simulink model "SegmentsDisplays"  (R2020b)
settings: Solver=FixedStepAuto  StartTime=0.0  StopTime=Inf  RelTol=1e-3  SampleTimeConstraint=STIndependent
undefined symbols (not defined in the file): DISPLAY_REGISTER_1, DISPLAY_REGISTER_2, DISPLAY_REGISTER_3
Description:
  | % Copyright 2019 The MathWorks, Inc.
settings Model: DataDictionary=Parameters.sldd  EnableAccessToBaseWorkspace=off  EnablePacing=on  Creator=sdupertu  LastModifiedBy=sebas
settings DataIOCC: SaveOutput=off  SaveTime=off
settings OptimizationCC: DefaultParameterBehavior=Inlined  EnhancedBackFolding=on  PassReuseOutputArgsAs=Individual arguments  OptimizeBlockOrder=speed  DifferentSizesBufferReuse=on  OptimizationCustomize=off  EfficientTunableParamExpr=on
settings DebuggingCC: ParameterTunabilityLossMsg=error  PregeneratedLibrarySubsystemCodeDiagnostic=none  ArithmeticOperatorsInVariantConditions=warning
settings ModelReferenceCC: EnableParallelModelReferenceBuilds=on
settings SFSimCC: SimUseLocalCustomCode=off  MATLABDynamicMemAlloc=off  CustomCodeUndefinedFunction=UseInterfaceOnly
settings RTWCC: Description=Embedded Coder  SystemTargetFile=ert.tlc  TemplateMakefile=ert_default_tmf  GenerateReport=on  RTWUseLocalCustomCode=off  IncludeHyperlinkInReport=on  LaunchReport=on  GenerateTraceInfo=on  GenerateTraceReport=on  GenerateTraceReportSl=on  GenerateTraceReportSf=on  GenerateTraceReportEml=on  GenerateWebview=on  GenerateCodeMetricsReport=on
settings CodeAppCC: ForceParamTrailComments=on  IgnoreCustomStorageClasses=off  MaxIdLength=61  OperatorAnnotations=on  SimulinkDataObjDesc=on  SFDataObjDesc=on  InsertBlockDesc=on
settings ERTTargetCC: TargetLangStandard=C99 (ISO)  GenerateSampleERTMain=on  InlinedParameterPlacement=NonHierarchical  ERTCustomFileTemplate=example_file_process.tlc

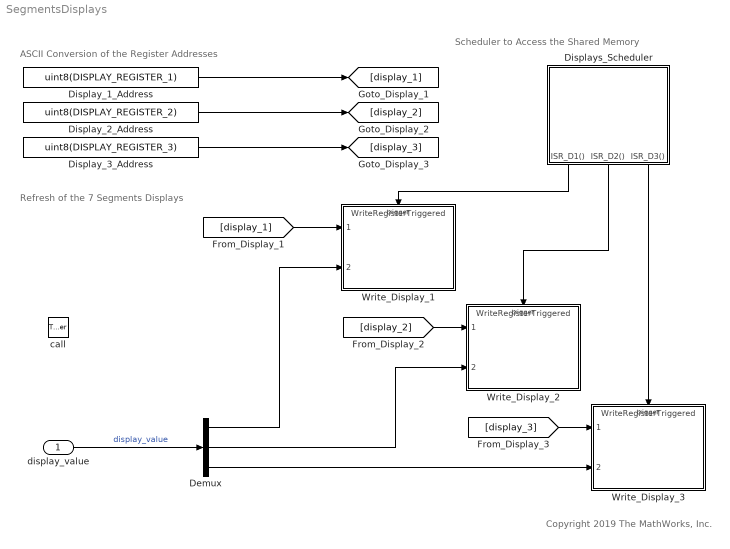
== system SegmentsDisplays ==
  note: Copyright 2019 The MathWorks, Inc.
  note: Scheduler to Access the Shared Memory
  note: Refresh of the 7 Segments Displays
  note: ASCII Conversion of the Register Addresses
  display_value : Inport  OutDataTypeStr=uint8  PortDimensions=[1 3]
  call : TriggerPort  TriggerType=function-call  VariantControl=Variant  SampleTime=-1  PortDimensions=1  TriggerSignalSampleTime=[0.001,0]
  Demux : Demux  Outputs=3
  Display_1_Address : Constant  Value=uint8(DISPLAY_REGISTER_1)  SampleTime=-1
  Display_2_Address : Constant  Value=uint8(DISPLAY_REGISTER_2)  SampleTime=-1
  Display_3_Address : Constant  Value=uint8(DISPLAY_REGISTER_3)  SampleTime=-1
  Displays_Scheduler : Stateflow chart  TreatAsAtomicUnit=on
  Write_Display_1 : ModelReference  ModelNameDialog=WriteRegisterTriggered  SimulationMode=Normal  ModelReferenceVersion=3.1  TriggerPortName=trigger  TriggerPortTriggerType=function-call  TriggerPortStatesWhenEnabling=held
  Write_Display_2 : ModelReference  ModelNameDialog=WriteRegisterTriggered  SimulationMode=Normal  ModelReferenceVersion=3.1  TriggerPortName=trigger  TriggerPortTriggerType=function-call  TriggerPortStatesWhenEnabling=held
  Write_Display_3 : ModelReference  ModelNameDialog=WriteRegisterTriggered  SimulationMode=Normal  ModelReferenceVersion=3.1  TriggerPortName=trigger  TriggerPortTriggerType=function-call  TriggerPortStatesWhenEnabling=held
  wires:
  Demux/2 -> Write_Display_2/2
  Demux/3 -> Write_Display_3/2
  Demux/1 -> Write_Display_1/2
  display_value/1 -> Demux/1  "display_value"
  Displays_Scheduler/1(ISR_D1()) -> Write_Display_1/Trigger
  Displays_Scheduler/2(ISR_D2()) -> Write_Display_2/Trigger
  Displays_Scheduler/3(ISR_D3()) -> Write_Display_3/Trigger
  Display_1_Address/1 -> [display_1]
  Display_2_Address/1 -> [display_2]
  Display_3_Address/1 -> [display_3]
  [display_1] -> Write_Display_1/1
  [display_2] -> Write_Display_2/1
  [display_3] -> Write_Display_3/1

== stateflow chart SegmentsDisplays/Displays_Scheduler ==
  state Update_DISP1
    entry: % Refresh the status of the first digits display
    send(ISR_D1);
  state Update_DISP2
    entry: % Refresh the status of the second digits display
    send(ISR_D2);
  state Update_DISP3
    entry: % Refresh the status of the third digits display
    send(ISR_D3);
  (default) -> Update_DISP1
  (junction 16) -> Update_DISP1
  (junction 17) -> (junction 16) : [after(2, tick)]
  Update_DISP1 -> Update_DISP2 : [after(2, tick)]
  Update_DISP2 -> Update_DISP3 : [after(2, tick)]
  Update_DISP3 -> (junction 17)
  events: ISR_D1 output FUNCTION_CALL_EVENT; ISR_D2 output FUNCTION_CALL_EVENT; ISR_D3 output FUNCTION_CALL_EVENT
